simulink model "multiroom_heating"  (R2022b)
settings: Solver=ode4  StartTime=0.0  StopTime=50  FixedStep=.001  RelTol=1e-3
libraries: simulink x1
settings Model: Creator=aryan  LastModifiedBy=aryan

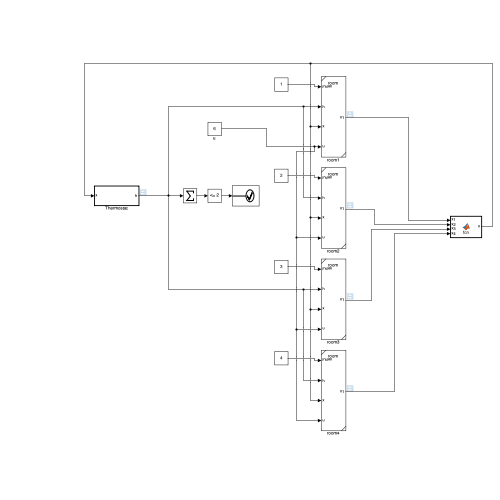
[thumbnail: Simulink's stored preview of the top-level diagram]
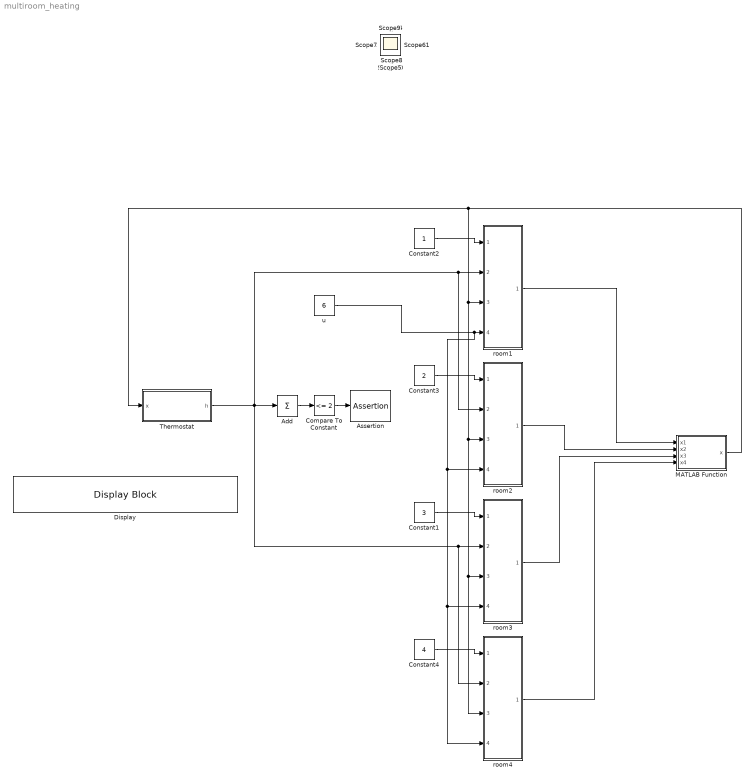
== system multiroom_heating ==
  Add : Sum  Inputs=+
  Assertion : Assertion  AssertionFailFcn="error(\"More than 2 heaters were turned on\")"
  Compare To Constant : simulink/Logic and Bit Operations/Compare To Constant  relop=<=  const=2  OutDataTypeStr=boolean
  Constant1 : Constant  Value=3
  Constant2 : Constant
  Constant3 : Constant  Value=2
  Constant4 : Constant  Value=4
  Display : DisplayBlock  LabelPosition=Hide  Transparency=1
  MATLAB Function : MATLAB Function  TreatAsAtomicUnit=on
  Thermostat : Subsystem  TreatAsAtomicUnit=on
  room{1..4} (4 alike) : Subsystem  ReferencedSubsystem=room
  u : Constant  Value=6
  Scope{,1..11} (12 alike) : Scope
  wires:
  Constant2/1 -> room1/1
  room1/1 -> MATLAB Function/1(x1)
  Constant3/1 -> room2/1
  Constant1/1 -> room3/1
  Constant4/1 -> room4/1
  room2/1 -> MATLAB Function/2(x2)
  room4/1 -> MATLAB Function/4(x4)
  room3/1 -> MATLAB Function/3(x3)
  u/1 -> room2/4, room3/4, room4/4, room1/4
  Thermostat/1(h) -> Add/1, room3/2, room4/2, room1/2, room2/2
  Add/1 -> Compare To Constant/1
  Compare To Constant/1 -> Assertion/1
  MATLAB Function/1(x) -> Thermostat/1(x), room4/3, room3/3, room2/3, room1/3

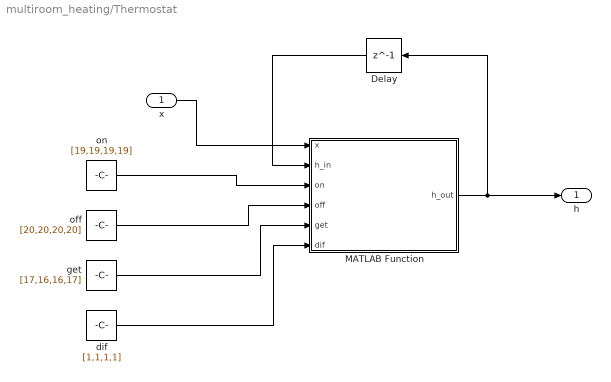
== system multiroom_heating/Thermostat ==
  x : Inport
  Delay : Delay  DelayLength=1  InitialCondition=[0,1,1,0]
  MATLAB Function : MATLAB Function  TreatAsAtomicUnit=on
  dif : Constant  Value=[1,1,1,1]
  get : Constant  Value=[17,16,16,17]
  off : Constant  Value=[20,20,20,20]
  on : Constant  Value=[19,19,19,19]
  h : Outport
  wires:
  on/1 -> MATLAB Function/3(on)
  off/1 -> MATLAB Function/4(off)
  get/1 -> MATLAB Function/5(get)
  dif/1 -> MATLAB Function/6(dif)
  MATLAB Function/1(h_out) -> Delay/1, h/1
  Delay/1 -> MATLAB Function/2(h_in)
  x/1 -> MATLAB Function/1(x)

== matlab function multiroom_heating/MATLAB Function ==
  data: x1 input; x output size=[1 4]; x2 input; x3 input; x4 input
function x = fcn(x1,x2,x3,x4)

x = [x1,x2,x3,x4];

== matlab function multiroom_heating/Thermostat/MATLAB Function ==
  data: x input; h_out output int8; h_in input int8 size=[1 4]; on input; off input; get input; dif input
function h_out    = fcn(x,h_in,on,off,get,dif)
% number of heaters
h_count = sum(h_in);
% maximum number of heaters allowed
MAX_HEATERS = 2;

% turn off heaters if necessary
for i = 1:4
    if h_in(i) == 1 && x(i) >= off(i)
        h_in(i) = 0;
        h_count = h_count - 1;
    end
end

% turn on heaters if necessary
for i = 1:4
    if h_in(i) == 0 && x(i) <= on(i) && h_count < MAX_HEATERS
        h_in(i) = 1;
        h_count = h_count + 1;
    end
end

% find the indices of the two heaters
h1 = -1;
h2 = -1;
for i = 1:4
    if h_in(i) == 1 && h1 == -1
        h1 = i;
    elseif h_in(i) == 1
        h2 = i;
    end
end

% move the first heater
% prioritize moving the heater to the coldest room
if h1 ~= -1
    min_temp = x(h1);
    min_idx = -1;
    for i = 1:4
        if (h_in(i) == 0) && (x(i) < get(i)) && (x(h1) - x(i) >= dif(i)) && (x(i) < min_temp)
            min_temp = x(i);
            min_idx = i;
        end
    end
    if min_idx ~= -1
        h_in(min_idx) = 1;
        h_in(h1) = 0;
    end
end

% move the second heater
if h2 ~= -1
    min_temp = x(h2);
    min_idx = -1;
    for i = 1:4
        if (h_in(i) == 0) && (x(i) < get(i)) && (x(h2) - x(i) >= dif(i)) && (x(i) < min_temp)
            min_temp = x(i);
            min_idx = i;
        end
    end
    if min_idx ~= -1
        h_in(min_idx) = 1;
        h_in(h2) = 0;
    end
end

h_out = h_in;
